simulink model "Oscillating"  (Simulink 8.5)
settings: Solver=ode45  StartTime=0.0  StopTime=tfinal  RelTol=1e-6
undefined symbols (not defined in the file): Ap, Bp, Cp, Dp, h, md
settings Model: Creator=jakesson  LastModifiedBy=jomle  ExtModeAutoUpdateStatusClock=off
settings DataIOCC: SignalLoggingName=sigsOut
settings OptimizationCC: BooleanDataType=off  ExpressionDepthLimit=128  InitFltsAndDblsToZero=on
settings DebuggingCC: SaveWithParameterizedLinksMsg=none  SignalResolutionControl=TryResolveAllWithWarning  MultiTaskDSMMsg=warning  MultiTaskCondExecSysMsg=none  FcnCallInpInsideContextMsg=UseLocalSettings  StateNameClashWarn=none
settings HardwareCC: TargetUnknown=on
settings GRTTargetCC: TargetFcnLib=ansi_tfl_tmw.mat

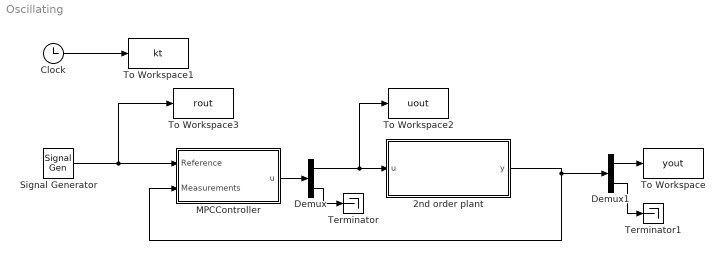
== system Oscillating ==
  2nd order plant : Subsystem
  Clock : Clock
  Demux : Demux  Outputs=[md.m md.ne]
  Demux1 : Demux  Outputs=2
  MPCController : Subsystem  mask{md=md}
      mask prompts: md "MPCData"
  Signal Generator : SignalGenerator  WaveForm=square  Frequency=0.05  Units=rad/sec
  Terminator : Terminator
  Terminator1 : Terminator
  To Workspace : ToWorkspace  VariableName=yout  SampleTime=-1
  To Workspace1 : ToWorkspace  VariableName=kt  SampleTime=-1
  To Workspace2 : ToWorkspace  VariableName=uout  SampleTime=-1
  To Workspace3 : ToWorkspace  VariableName=rout  SampleTime=-1
  wires:
  2nd order plant/1(y) -> Demux1/1, MPCController/2(Measurements)
  Demux/2 -> Terminator/1
  MPCController/1(u) -> Demux/1
  Clock/1 -> To Workspace1/1
  Demux/1 -> 2nd order plant/1(u), To Workspace2/1
  Signal Generator/1 -> To Workspace3/1, MPCController/1(Reference)
  Demux1/2 -> Terminator1/1
  Demux1/1 -> To Workspace/1

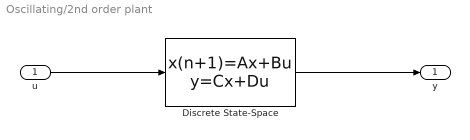
== system Oscillating/2nd order plant ==
  u : Inport
  Discrete State-Space : DiscreteStateSpace  A=Ap  B=Bp  C=Cp  D=Dp  SampleTime=h
  y : Outport
  wires:
  Discrete State-Space/1 -> y/1
  u/1 -> Discrete State-Space/1

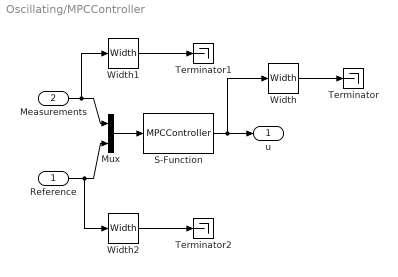
== system Oscillating/MPCController ==
  Reference : Inport
  Measurements : Inport  Port=2
  Mux : Mux  Inputs=2
  S-Function : S-Function  FunctionName=MPCController  Parameters=md
  Terminator : Terminator
  Terminator1 : Terminator
  Terminator2 : Terminator
  Width : Width
  Width1 : Width
  Width2 : Width
  u : Outport
  wires:
  Mux/1 -> S-Function/1
  Measurements/1 -> Width1/1, Mux/1
  Reference/1 -> Width2/1, Mux/2
  S-Function/1 -> Width/1, u/1
  Width/1 -> Terminator/1
  Width1/1 -> Terminator1/1
  Width2/1 -> Terminator2/1
